simulink model "simulation17PDfract"  (R2025b)
settings: Solver=ode45  StartTime=0.0  StopTime=0.5  FixedStep=h  RelTol=1e-9
values from neighbouring files (symbols this model uses):
  h = 0.001    [run_3d_simbody_suite.m]    (also in run_all_simulations.m)
  kd = 1.0245    [run_3d_simbody_suite.m]
  kp = 16    [run_3d_simbody_suite.m]
  mu = 0.5308    [run_3d_simbody_suite.m]
  n = double(ceil(tf/h))    [run_3d_simbody_suite.m]    (also in run_all_simulations.m)
undefined symbols (not defined in the file or in its folder): X, Y, Z
libraries: sm_lib x327, nesl_utility x14, simulink x7, fod x3, checkpacklib x1
(part 8 of 8)

== system simulation17PDfract/RD_SM2/BrasParalelle1/BarreParalleles_2_RIGID/Pice4_Extremetees_1_RIGID ==
  ReferenceFrame : sm_lib/Frames and Transforms/Reference Frame
  Solid : sm_lib/Body Elements/File Solid  ExtGeomFileName=Pièce4_Extremetees_Défaut_sldprt.STL  UnitType=Custom  ExtGeomFileUnits=mm  StepReaderType=HEX  ExportConvexHullGeometry=off  InertiaType=Custom  Mass=0.0043409919402835973  MassUnits=kg  CenterOfMass=[-6.6394731011390018e-06 -1.3723999560385911 4.9969803448403587]  CenterOfMassUnits=mm  MomentsOfInertia=[0.22208105944838133 0.24049053699814107 0.066049415613599144]  MomentsOfInertiaUnits=kg*mm^2  ProductsOfInertia=[-0.022728057317176146 1.1398156711642886e-07 7.9844492116922665e-07]  ProductsOfInertiaUnits=kg*mm^2  BasedOnType=Density  Density=1000  DensityUnits=kg/(m^3)  DoExposeReferenceFrame=on  SerializedFrames=<Frames/>  GraphicType=FromGeometry  MarkerShape=Sphere  MarkerSize=10  MarkerSizeUnits=m  GraphicVisPropType=SimpleVisualProperties  GraphicDiffuseColor=[0.59999999999999998 0.59999999999999998 0.59999999999999998]  GraphicSpecularColor=[0.5 0.5 0.5 1.0]  GraphicAmbientColor=[0.15 0.15 0.15 1.0]  GraphicEmissiveColor=[0.0 0.0 0.0 1.0]  GraphicShininess=75  GraphicOpacity=1
  F : PMIOPort  Side=Left
  connections:
  Solid/RConn1 -- ReferenceFrame/RConn1 -- F/RConn1

== system simulation17PDfract/RD_SM2/BrasParalelle1/BarreParalleles_2_RIGID/Pice4_Extremetees_2_RIGID ==
  ReferenceFrame : sm_lib/Frames and Transforms/Reference Frame
  Solid : sm_lib/Body Elements/File Solid  ExtGeomFileName=Pièce4_Extremetees_Défaut_sldprt.STL  UnitType=Custom  ExtGeomFileUnits=mm  StepReaderType=HEX  ExportConvexHullGeometry=off  InertiaType=Custom  Mass=0.0043409919402835973  MassUnits=kg  CenterOfMass=[-6.6394731011390018e-06 -1.3723999560385911 4.9969803448403587]  CenterOfMassUnits=mm  MomentsOfInertia=[0.22208105944838133 0.24049053699814107 0.066049415613599144]  MomentsOfInertiaUnits=kg*mm^2  ProductsOfInertia=[-0.022728057317176146 1.1398156711642886e-07 7.9844492116922665e-07]  ProductsOfInertiaUnits=kg*mm^2  BasedOnType=Density  Density=1000  DensityUnits=kg/(m^3)  DoExposeReferenceFrame=on  SerializedFrames=<Frames/>  GraphicType=FromGeometry  MarkerShape=Sphere  MarkerSize=10  MarkerSizeUnits=m  GraphicVisPropType=SimpleVisualProperties  GraphicDiffuseColor=[0.59999999999999998 0.59999999999999998 0.59999999999999998]  GraphicSpecularColor=[0.5 0.5 0.5 1.0]  GraphicAmbientColor=[0.15 0.15 0.15 1.0]  GraphicEmissiveColor=[0.0 0.0 0.0 1.0]  GraphicShininess=75  GraphicOpacity=1
  F : PMIOPort  Side=Left
  connections:
  Solid/RConn1 -- ReferenceFrame/RConn1 -- F/RConn1

== system simulation17PDfract/RD_SM2/BrasParalelle1/BarreParalleles_2_RIGID/Pice4_Tube_1_RIGID ==
  ReferenceFrame : sm_lib/Frames and Transforms/Reference Frame
  Solid : sm_lib/Body Elements/File Solid  ExtGeomFileName=Pièce4_Tube_Défaut_sldprt.STL  UnitType=Custom  ExtGeomFileUnits=mm  StepReaderType=HEX  ExportConvexHullGeometry=off  InertiaType=Custom  Mass=0.0056953775725032503  MassUnits=kg  CenterOfMass=[-4.1460122344799134e-11 2.6332345173922464e-08 157.00037492761294]  CenterOfMassUnits=mm  MomentsOfInertia=[46.656669534748204 46.656784060773653 0.060513437161415502]  MomentsOfInertiaUnits=kg*mm^2  ProductsOfInertia=[4.4271388779002391e-06 -1.0344554341986986e-06 -6.5578304138838094e-07]  ProductsOfInertiaUnits=kg*mm^2  BasedOnType=Density  Density=1000  DensityUnits=kg/(m^3)  DoExposeReferenceFrame=on  SerializedFrames=<Frames/>  GraphicType=FromGeometry  MarkerShape=Sphere  MarkerSize=10  MarkerSizeUnits=m  GraphicVisPropType=SimpleVisualProperties  GraphicDiffuseColor=[1 1 1]  GraphicSpecularColor=[0.5 0.5 0.5 1.0]  GraphicAmbientColor=[0.15 0.15 0.15 1.0]  GraphicEmissiveColor=[0.0 0.0 0.0 1.0]  GraphicShininess=75  GraphicOpacity=1
  F : PMIOPort  Side=Left
  connections:
  Solid/RConn1 -- ReferenceFrame/RConn1 -- F/RConn1

== system simulation17PDfract/RD_SM2/BrasParalelle2/BarreParalleles_1_RIGID/Pice4_Extremetees_1_RIGID ==
  ReferenceFrame : sm_lib/Frames and Transforms/Reference Frame
  Solid : sm_lib/Body Elements/File Solid  ExtGeomFileName=Pièce4_Extremetees_Défaut_sldprt.STL  UnitType=Custom  ExtGeomFileUnits=mm  StepReaderType=HEX  ExportConvexHullGeometry=off  InertiaType=Custom  Mass=0.0043409919402835973  MassUnits=kg  CenterOfMass=[-6.6394731011390018e-06 -1.3723999560385911 4.9969803448403587]  CenterOfMassUnits=mm  MomentsOfInertia=[0.22208105944838133 0.24049053699814107 0.066049415613599144]  MomentsOfInertiaUnits=kg*mm^2  ProductsOfInertia=[-0.022728057317176146 1.1398156711642886e-07 7.9844492116922665e-07]  ProductsOfInertiaUnits=kg*mm^2  BasedOnType=Density  Density=1000  DensityUnits=kg/(m^3)  DoExposeReferenceFrame=on  SerializedFrames=<Frames/>  GraphicType=FromGeometry  MarkerShape=Sphere  MarkerSize=10  MarkerSizeUnits=m  GraphicVisPropType=SimpleVisualProperties  GraphicDiffuseColor=[0.59999999999999998 0.59999999999999998 0.59999999999999998]  GraphicSpecularColor=[0.5 0.5 0.5 1.0]  GraphicAmbientColor=[0.15 0.15 0.15 1.0]  GraphicEmissiveColor=[0.0 0.0 0.0 1.0]  GraphicShininess=75  GraphicOpacity=1
  F : PMIOPort  Side=Left
  connections:
  F/RConn1 -- ReferenceFrame/RConn1 -- Solid/RConn1

== system simulation17PDfract/RD_SM2/BrasParalelle2/BarreParalleles_1_RIGID/Pice4_Extremetees_2_RIGID ==
  ReferenceFrame : sm_lib/Frames and Transforms/Reference Frame
  Solid : sm_lib/Body Elements/File Solid  ExtGeomFileName=Pièce4_Extremetees_Défaut_sldprt.STL  UnitType=Custom  ExtGeomFileUnits=mm  StepReaderType=HEX  ExportConvexHullGeometry=off  InertiaType=Custom  Mass=0.0043409919402835973  MassUnits=kg  CenterOfMass=[-6.6394731011390018e-06 -1.3723999560385911 4.9969803448403587]  CenterOfMassUnits=mm  MomentsOfInertia=[0.22208105944838133 0.24049053699814107 0.066049415613599144]  MomentsOfInertiaUnits=kg*mm^2  ProductsOfInertia=[-0.022728057317176146 1.1398156711642886e-07 7.9844492116922665e-07]  ProductsOfInertiaUnits=kg*mm^2  BasedOnType=Density  Density=1000  DensityUnits=kg/(m^3)  DoExposeReferenceFrame=on  SerializedFrames=<Frames/>  GraphicType=FromGeometry  MarkerShape=Sphere  MarkerSize=10  MarkerSizeUnits=m  GraphicVisPropType=SimpleVisualProperties  GraphicDiffuseColor=[0.59999999999999998 0.59999999999999998 0.59999999999999998]  GraphicSpecularColor=[0.5 0.5 0.5 1.0]  GraphicAmbientColor=[0.15 0.15 0.15 1.0]  GraphicEmissiveColor=[0.0 0.0 0.0 1.0]  GraphicShininess=75  GraphicOpacity=1
  F : PMIOPort  Side=Left
  connections:
  F/RConn1 -- ReferenceFrame/RConn1 -- Solid/RConn1

== system simulation17PDfract/RD_SM2/BrasParalelle2/BarreParalleles_1_RIGID/Pice4_Tube_1_RIGID ==
  ReferenceFrame : sm_lib/Frames and Transforms/Reference Frame
  Solid : sm_lib/Body Elements/File Solid  ExtGeomFileName=Pièce4_Tube_Défaut_sldprt.STL  UnitType=Custom  ExtGeomFileUnits=mm  StepReaderType=HEX  ExportConvexHullGeometry=off  InertiaType=Custom  Mass=0.0056953775725032503  MassUnits=kg  CenterOfMass=[-4.1460122344799134e-11 2.6332345173922464e-08 157.00037492761294]  CenterOfMassUnits=mm  MomentsOfInertia=[46.656669534748204 46.656784060773653 0.060513437161415502]  MomentsOfInertiaUnits=kg*mm^2  ProductsOfInertia=[4.4271388779002391e-06 -1.0344554341986986e-06 -6.5578304138838094e-07]  ProductsOfInertiaUnits=kg*mm^2  BasedOnType=Density  Density=1000  DensityUnits=kg/(m^3)  DoExposeReferenceFrame=on  SerializedFrames=<Frames/>  GraphicType=FromGeometry  MarkerShape=Sphere  MarkerSize=10  MarkerSizeUnits=m  GraphicVisPropType=SimpleVisualProperties  GraphicDiffuseColor=[1 1 1]  GraphicSpecularColor=[0.5 0.5 0.5 1.0]  GraphicAmbientColor=[0.15 0.15 0.15 1.0]  GraphicEmissiveColor=[0.0 0.0 0.0 1.0]  GraphicShininess=75  GraphicOpacity=1
  F : PMIOPort  Side=Left
  connections:
  F/RConn1 -- ReferenceFrame/RConn1 -- Solid/RConn1

== system simulation17PDfract/RD_SM2/BrasParalelle2/BarreParalleles_2_RIGID/Pice4_Extremetees_1_RIGID ==
  ReferenceFrame : sm_lib/Frames and Transforms/Reference Frame
  Solid : sm_lib/Body Elements/File Solid  ExtGeomFileName=Pièce4_Extremetees_Défaut_sldprt.STL  UnitType=Custom  ExtGeomFileUnits=mm  StepReaderType=HEX  ExportConvexHullGeometry=off  InertiaType=Custom  Mass=0.0043409919402835973  MassUnits=kg  CenterOfMass=[-6.6394731011390018e-06 -1.3723999560385911 4.9969803448403587]  CenterOfMassUnits=mm  MomentsOfInertia=[0.22208105944838133 0.24049053699814107 0.066049415613599144]  MomentsOfInertiaUnits=kg*mm^2  ProductsOfInertia=[-0.022728057317176146 1.1398156711642886e-07 7.9844492116922665e-07]  ProductsOfInertiaUnits=kg*mm^2  BasedOnType=Density  Density=1000  DensityUnits=kg/(m^3)  DoExposeReferenceFrame=on  SerializedFrames=<Frames/>  GraphicType=FromGeometry  MarkerShape=Sphere  MarkerSize=10  MarkerSizeUnits=m  GraphicVisPropType=SimpleVisualProperties  GraphicDiffuseColor=[0.59999999999999998 0.59999999999999998 0.59999999999999998]  GraphicSpecularColor=[0.5 0.5 0.5 1.0]  GraphicAmbientColor=[0.15 0.15 0.15 1.0]  GraphicEmissiveColor=[0.0 0.0 0.0 1.0]  GraphicShininess=75  GraphicOpacity=1
  F : PMIOPort  Side=Left
  connections:
  F/RConn1 -- ReferenceFrame/RConn1 -- Solid/RConn1

== system simulation17PDfract/RD_SM2/BrasParalelle2/BarreParalleles_2_RIGID/Pice4_Extremetees_2_RIGID ==
  ReferenceFrame : sm_lib/Frames and Transforms/Reference Frame
  Solid : sm_lib/Body Elements/File Solid  ExtGeomFileName=Pièce4_Extremetees_Défaut_sldprt.STL  UnitType=Custom  ExtGeomFileUnits=mm  StepReaderType=HEX  ExportConvexHullGeometry=off  InertiaType=Custom  Mass=0.0043409919402835973  MassUnits=kg  CenterOfMass=[-6.6394731011390018e-06 -1.3723999560385911 4.9969803448403587]  CenterOfMassUnits=mm  MomentsOfInertia=[0.22208105944838133 0.24049053699814107 0.066049415613599144]  MomentsOfInertiaUnits=kg*mm^2  ProductsOfInertia=[-0.022728057317176146 1.1398156711642886e-07 7.9844492116922665e-07]  ProductsOfInertiaUnits=kg*mm^2  BasedOnType=Density  Density=1000  DensityUnits=kg/(m^3)  DoExposeReferenceFrame=on  SerializedFrames=<Frames/>  GraphicType=FromGeometry  MarkerShape=Sphere  MarkerSize=10  MarkerSizeUnits=m  GraphicVisPropType=SimpleVisualProperties  GraphicDiffuseColor=[0.59999999999999998 0.59999999999999998 0.59999999999999998]  GraphicSpecularColor=[0.5 0.5 0.5 1.0]  GraphicAmbientColor=[0.15 0.15 0.15 1.0]  GraphicEmissiveColor=[0.0 0.0 0.0 1.0]  GraphicShininess=75  GraphicOpacity=1
  F : PMIOPort  Side=Left
  connections:
  F/RConn1 -- ReferenceFrame/RConn1 -- Solid/RConn1

== system simulation17PDfract/RD_SM2/BrasParalelle2/BarreParalleles_2_RIGID/Pice4_Tube_1_RIGID ==
  ReferenceFrame : sm_lib/Frames and Transforms/Reference Frame
  Solid : sm_lib/Body Elements/File Solid  ExtGeomFileName=Pièce4_Tube_Défaut_sldprt.STL  UnitType=Custom  ExtGeomFileUnits=mm  StepReaderType=HEX  ExportConvexHullGeometry=off  InertiaType=Custom  Mass=0.0056953775725032503  MassUnits=kg  CenterOfMass=[-4.1460122344799134e-11 2.6332345173922464e-08 157.00037492761294]  CenterOfMassUnits=mm  MomentsOfInertia=[46.656669534748204 46.656784060773653 0.060513437161415502]  MomentsOfInertiaUnits=kg*mm^2  ProductsOfInertia=[4.4271388779002391e-06 -1.0344554341986986e-06 -6.5578304138838094e-07]  ProductsOfInertiaUnits=kg*mm^2  BasedOnType=Density  Density=1000  DensityUnits=kg/(m^3)  DoExposeReferenceFrame=on  SerializedFrames=<Frames/>  GraphicType=FromGeometry  MarkerShape=Sphere  MarkerSize=10  MarkerSizeUnits=m  GraphicVisPropType=SimpleVisualProperties  GraphicDiffuseColor=[1 1 1]  GraphicSpecularColor=[0.5 0.5 0.5 1.0]  GraphicAmbientColor=[0.15 0.15 0.15 1.0]  GraphicEmissiveColor=[0.0 0.0 0.0 1.0]  GraphicShininess=75  GraphicOpacity=1
  F : PMIOPort  Side=Left
  connections:
  F/RConn1 -- ReferenceFrame/RConn1 -- Solid/RConn1

== system simulation17PDfract/RD_SM2/BrasParalelle3/BarreParalleles_1_RIGID/Pice4_Extremetees_1_RIGID ==
  ReferenceFrame : sm_lib/Frames and Transforms/Reference Frame
  Solid : sm_lib/Body Elements/File Solid  ExtGeomFileName=Pièce4_Extremetees_Défaut_sldprt.STL  UnitType=Custom  ExtGeomFileUnits=mm  StepReaderType=HEX  ExportConvexHullGeometry=off  InertiaType=Custom  Mass=0.0043409919402835973  MassUnits=kg  CenterOfMass=[-6.6394731011390018e-06 -1.3723999560385911 4.9969803448403587]  CenterOfMassUnits=mm  MomentsOfInertia=[0.22208105944838133 0.24049053699814107 0.066049415613599144]  MomentsOfInertiaUnits=kg*mm^2  ProductsOfInertia=[-0.022728057317176146 1.1398156711642886e-07 7.9844492116922665e-07]  ProductsOfInertiaUnits=kg*mm^2  BasedOnType=Density  Density=1000  DensityUnits=kg/(m^3)  DoExposeReferenceFrame=on  SerializedFrames=<Frames/>  GraphicType=FromGeometry  MarkerShape=Sphere  MarkerSize=10  MarkerSizeUnits=m  GraphicVisPropType=SimpleVisualProperties  GraphicDiffuseColor=[0.59999999999999998 0.59999999999999998 0.59999999999999998]  GraphicSpecularColor=[0.5 0.5 0.5 1.0]  GraphicAmbientColor=[0.15 0.15 0.15 1.0]  GraphicEmissiveColor=[0.0 0.0 0.0 1.0]  GraphicShininess=75  GraphicOpacity=1
  F : PMIOPort  Side=Left
  connections:
  Solid/RConn1 -- ReferenceFrame/RConn1 -- F/RConn1

== system simulation17PDfract/RD_SM2/BrasParalelle3/BarreParalleles_1_RIGID/Pice4_Extremetees_2_RIGID ==
  ReferenceFrame : sm_lib/Frames and Transforms/Reference Frame
  Solid : sm_lib/Body Elements/File Solid  ExtGeomFileName=Pièce4_Extremetees_Défaut_sldprt.STL  UnitType=Custom  ExtGeomFileUnits=mm  StepReaderType=HEX  ExportConvexHullGeometry=off  InertiaType=Custom  Mass=0.0043409919402835973  MassUnits=kg  CenterOfMass=[-6.6394731011390018e-06 -1.3723999560385911 4.9969803448403587]  CenterOfMassUnits=mm  MomentsOfInertia=[0.22208105944838133 0.24049053699814107 0.066049415613599144]  MomentsOfInertiaUnits=kg*mm^2  ProductsOfInertia=[-0.022728057317176146 1.1398156711642886e-07 7.9844492116922665e-07]  ProductsOfInertiaUnits=kg*mm^2  BasedOnType=Density  Density=1000  DensityUnits=kg/(m^3)  DoExposeReferenceFrame=on  SerializedFrames=<Frames/>  GraphicType=FromGeometry  MarkerShape=Sphere  MarkerSize=10  MarkerSizeUnits=m  GraphicVisPropType=SimpleVisualProperties  GraphicDiffuseColor=[0.59999999999999998 0.59999999999999998 0.59999999999999998]  GraphicSpecularColor=[0.5 0.5 0.5 1.0]  GraphicAmbientColor=[0.15 0.15 0.15 1.0]  GraphicEmissiveColor=[0.0 0.0 0.0 1.0]  GraphicShininess=75  GraphicOpacity=1
  F : PMIOPort  Side=Left
  connections:
  Solid/RConn1 -- ReferenceFrame/RConn1 -- F/RConn1

== system simulation17PDfract/RD_SM2/BrasParalelle3/BarreParalleles_1_RIGID/Pice4_Tube_1_RIGID ==
  ReferenceFrame : sm_lib/Frames and Transforms/Reference Frame
  Solid : sm_lib/Body Elements/File Solid  ExtGeomFileName=Pièce4_Tube_Défaut_sldprt.STL  UnitType=Custom  ExtGeomFileUnits=mm  StepReaderType=HEX  ExportConvexHullGeometry=off  InertiaType=Custom  Mass=0.0056953775725032503  MassUnits=kg  CenterOfMass=[-4.1460122344799134e-11 2.6332345173922464e-08 157.00037492761294]  CenterOfMassUnits=mm  MomentsOfInertia=[46.656669534748204 46.656784060773653 0.060513437161415502]  MomentsOfInertiaUnits=kg*mm^2  ProductsOfInertia=[4.4271388779002391e-06 -1.0344554341986986e-06 -6.5578304138838094e-07]  ProductsOfInertiaUnits=kg*mm^2  BasedOnType=Density  Density=1000  DensityUnits=kg/(m^3)  DoExposeReferenceFrame=on  SerializedFrames=<Frames/>  GraphicType=FromGeometry  MarkerShape=Sphere  MarkerSize=10  MarkerSizeUnits=m  GraphicVisPropType=SimpleVisualProperties  GraphicDiffuseColor=[1 1 1]  GraphicSpecularColor=[0.5 0.5 0.5 1.0]  GraphicAmbientColor=[0.15 0.15 0.15 1.0]  GraphicEmissiveColor=[0.0 0.0 0.0 1.0]  GraphicShininess=75  GraphicOpacity=1
  F : PMIOPort  Side=Left
  connections:
  Solid/RConn1 -- ReferenceFrame/RConn1 -- F/RConn1

== system simulation17PDfract/RD_SM2/BrasParalelle3/BarreParalleles_2_RIGID/Pice4_Extremetees_1_RIGID ==
  ReferenceFrame : sm_lib/Frames and Transforms/Reference Frame
  Solid : sm_lib/Body Elements/File Solid  ExtGeomFileName=Pièce4_Extremetees_Défaut_sldprt.STL  UnitType=Custom  ExtGeomFileUnits=mm  StepReaderType=HEX  ExportConvexHullGeometry=off  InertiaType=Custom  Mass=0.0043409919402835973  MassUnits=kg  CenterOfMass=[-6.6394731011390018e-06 -1.3723999560385911 4.9969803448403587]  CenterOfMassUnits=mm  MomentsOfInertia=[0.22208105944838133 0.24049053699814107 0.066049415613599144]  MomentsOfInertiaUnits=kg*mm^2  ProductsOfInertia=[-0.022728057317176146 1.1398156711642886e-07 7.9844492116922665e-07]  ProductsOfInertiaUnits=kg*mm^2  BasedOnType=Density  Density=1000  DensityUnits=kg/(m^3)  DoExposeReferenceFrame=on  SerializedFrames=<Frames/>  GraphicType=FromGeometry  MarkerShape=Sphere  MarkerSize=10  MarkerSizeUnits=m  GraphicVisPropType=SimpleVisualProperties  GraphicDiffuseColor=[0.59999999999999998 0.59999999999999998 0.59999999999999998]  GraphicSpecularColor=[0.5 0.5 0.5 1.0]  GraphicAmbientColor=[0.15 0.15 0.15 1.0]  GraphicEmissiveColor=[0.0 0.0 0.0 1.0]  GraphicShininess=75  GraphicOpacity=1
  F : PMIOPort  Side=Left
  connections:
  Solid/RConn1 -- ReferenceFrame/RConn1 -- F/RConn1

== system simulation17PDfract/RD_SM2/BrasParalelle3/BarreParalleles_2_RIGID/Pice4_Extremetees_2_RIGID ==
  ReferenceFrame : sm_lib/Frames and Transforms/Reference Frame
  Solid : sm_lib/Body Elements/File Solid  ExtGeomFileName=Pièce4_Extremetees_Défaut_sldprt.STL  UnitType=Custom  ExtGeomFileUnits=mm  StepReaderType=HEX  ExportConvexHullGeometry=off  InertiaType=Custom  Mass=0.0043409919402835973  MassUnits=kg  CenterOfMass=[-6.6394731011390018e-06 -1.3723999560385911 4.9969803448403587]  CenterOfMassUnits=mm  MomentsOfInertia=[0.22208105944838133 0.24049053699814107 0.066049415613599144]  MomentsOfInertiaUnits=kg*mm^2  ProductsOfInertia=[-0.022728057317176146 1.1398156711642886e-07 7.9844492116922665e-07]  ProductsOfInertiaUnits=kg*mm^2  BasedOnType=Density  Density=1000  DensityUnits=kg/(m^3)  DoExposeReferenceFrame=on  SerializedFrames=<Frames/>  GraphicType=FromGeometry  MarkerShape=Sphere  MarkerSize=10  MarkerSizeUnits=m  GraphicVisPropType=SimpleVisualProperties  GraphicDiffuseColor=[0.59999999999999998 0.59999999999999998 0.59999999999999998]  GraphicSpecularColor=[0.5 0.5 0.5 1.0]  GraphicAmbientColor=[0.15 0.15 0.15 1.0]  GraphicEmissiveColor=[0.0 0.0 0.0 1.0]  GraphicShininess=75  GraphicOpacity=1
  F : PMIOPort  Side=Left
  connections:
  Solid/RConn1 -- ReferenceFrame/RConn1 -- F/RConn1

== system simulation17PDfract/RD_SM2/BrasParalelle3/BarreParalleles_2_RIGID/Pice4_Tube_1_RIGID ==
  ReferenceFrame : sm_lib/Frames and Transforms/Reference Frame
  Solid : sm_lib/Body Elements/File Solid  ExtGeomFileName=Pièce4_Tube_Défaut_sldprt.STL  UnitType=Custom  ExtGeomFileUnits=mm  StepReaderType=HEX  ExportConvexHullGeometry=off  InertiaType=Custom  Mass=0.0056953775725032503  MassUnits=kg  CenterOfMass=[-4.1460122344799134e-11 2.6332345173922464e-08 157.00037492761294]  CenterOfMassUnits=mm  MomentsOfInertia=[46.656669534748204 46.656784060773653 0.060513437161415502]  MomentsOfInertiaUnits=kg*mm^2  ProductsOfInertia=[4.4271388779002391e-06 -1.0344554341986986e-06 -6.5578304138838094e-07]  ProductsOfInertiaUnits=kg*mm^2  BasedOnType=Density  Density=1000  DensityUnits=kg/(m^3)  DoExposeReferenceFrame=on  SerializedFrames=<Frames/>  GraphicType=FromGeometry  MarkerShape=Sphere  MarkerSize=10  MarkerSizeUnits=m  GraphicVisPropType=SimpleVisualProperties  GraphicDiffuseColor=[1 1 1]  GraphicSpecularColor=[0.5 0.5 0.5 1.0]  GraphicAmbientColor=[0.15 0.15 0.15 1.0]  GraphicEmissiveColor=[0.0 0.0 0.0 1.0]  GraphicShininess=75  GraphicOpacity=1
  F : PMIOPort  Side=Left
  connections:
  Solid/RConn1 -- ReferenceFrame/RConn1 -- F/RConn1

== matlab function simulation17PDfract/fract PID2/frac_deriv/MATLAB Function ==
  data: u1 input; u2 input; u3 input; df output; clock input; q input; h input; n input
function df  = fcn(u1,u2,u3,clock,q,h,n)

df1 = 0;
df2 = 0;
df3 = 0;


cqj = zeros(1,501);

j = ceil(clock/h);
cqj(1,1) = 1;

for i = 1:j
    
    if i~=1
        cqj(i) = cqj(i-1)*(1-(1+q)/(i-1));
    end

    df1 = df1+h^-q*cqj(i)*u1(i);
    df2 = df2+h^-q*cqj(i)*u2(i);
    df3 = df3+h^-q*cqj(i)*u3(i);
end

df = [df1 df2 df3];

== matlab function simulation17PDfract/MATLAB Function6 ==
  data: P input; x output; y output; z output
function [x,y,z] = demux(P)
x = P(1,1);
y = P(1,2);
z = P(1,3);

== matlab function simulation17PDfract/RD_SM2/adaptation ==
  data: alpha input; Theta output; dalpha input; dTheta output
function [Theta,dTheta]= fcn(alpha,dalpha)
%RQ : l'angle alpha est decalee de shift = -0.0651 red (problemme simmechanics)
Theta = -12*(alpha - 0.0651*[1;1;1]) ;
dTheta = -12*dalpha ;

== matlab function simulation17PDfract/trajectoire/MATLAB Function1 ==
  data: P output; p input; t input; dP output; ddP output
function [P,dP,ddP]  = trajectoire(p,t)


A=0.25;
B=0.06;
D=pi*sqrt((A^2+B^2)/2);



Xdes=0.25-A*(1-cos(pi*(t)/(p*D)));
Ydes=0*t;
Zdes=-0.43+B*sin(pi*(t)/(p*D));

dXdes=-A*pi/(p*D)*(sin(pi*(t)/(p*D)));
dYdes=0*t;
dZdes=B*pi/(p*D)*cos(pi*(t)/(p*D));

ddXdes=A*pi/(p*D)*pi/(p*D)*cos(pi*(t)/(p*D));
ddYdes=0*t;
ddZdes=-B*pi/(p*D)*pi/(p*D)*sin(pi*(t)/(p*D));

% Xdes=-0.25+A*(1-cos(pi*t/(p*D)));
% Ydes=0*t;
% Zdes=-0.43+B*sin(pi*t/(p*D));

P = [Xdes,Ydes,Zdes];
dP = [dXdes,dYdes,dZdes];
ddP = [ddXdes,ddYdes,ddZdes];

end

== matlab function simulation17PDfract/MATLAB Function ==
  data: alpha input; P output; data input
function P  = MGD(alpha, data)

phi = [0 2*pi/3 4*pi/3];
l1 = 0.205;
l2 = 0.380;
r = 0.15-0.024;

D = zeros(1,3);
E = zeros(1,3);
F = zeros(1,3);
G = zeros(1,3);

for i=1:3
   D(i)=-l2^2+l1^2+r^2+2*r*l1*cos(alpha(i));
   E(i)=2*(r+l1*cos(alpha(i)))*cos(phi(i));
   F(i)=2*(r+l1*cos(alpha(i)))*sin(phi(i));
   G(i)=-2*l1*sin(alpha(i))  ;
end
% H1 = -(E(3)-E(1))*(G(2)-G(1))+(G(3)-G(1))*(E(2)-E(1));
% H2 = -(F(3)-F(1))*(E(2)-E(1))+(E(3)-E(1))*(F(2)-F(1));
% H3 = -(D(3)-D(1))*(E(2)-E(1))+(E(3)-E(1))*(D(2)-D(1));
% H4 = (D(3)-D(1))*(F(2)-F(1))-(F(3)-F(1))*(D(1)-D(2));
% H5 = -(G(3)-G(1))*(F(2)-F(1))-(F(3)-F(1))*(G(1)-G(2));

H1 = E(1)*G(2)-E(1)*G(3)-E(2)*G(1)+E(2)*G(3)+E(3)*G(1)-E(3)*G(2);
H2 = E(1)*(-F(2)+F(3))+E(2)*(F(1)-F(3))+E(3)*(-F(1)+F(2));
H3 = E(1)*(-D(2)+D(3))+E(2)*(D(1)-D(3))+E(3)*(-D(1)+D(2));
H4 = F(1)*(D(2)-D(3))+F(2)*(-D(1)+D(3))+F(3)*(D(1)-D(2));
H5 = F(1)*(-G(2)+G(3))+F(2)*(G(1)-G(3))+F(3)*(-G(1)+G(2));

L = ((H5^2+H1^2)/(H2^2))+1;
M = 2*(H5*H4+H1*H3)/(H2^2)-(H5*E(1)+H1*F(1))/H2-G(1);
N = (H4^2+H3^2)/H2^2-(H4*E(1)+H3*F(1))/H2+D(1);
Z = min((-M+sqrt(abs(M^2-4*L*N)))/(2*L),(-M-sqrt(abs(M^2-4*L*N)))/(2*L));
X = Z*(H5/H2)+(H4/H2);
Y = Z*(H1/H2)+(H3/H2);

X = double(X);
Y = double(Y);
Z = double(Z);

P = [X,Y,Z];

== matlab function simulation17PDfract/model inverse/MATLAB Function4 ==
  data: alpha input; ddalpha output; dalpha input; P input; dP input; ddP input
function ddalpha = MAI(alpha,dalpha,P,dP,ddP)

phi = [0 2*pi/3 4*pi/3];
l1 = 0.205;
r = 0.15-0.024;

% documentation 0

% rotation matrix
R1 = [cos(phi(1)) -sin(phi(1)) 0;sin(phi(1)) cos(phi(1)) 0;0 0 1];
R2 = [cos(phi(2)) -sin(phi(2)) 0;sin(phi(2)) cos(phi(2)) 0;0 0 1]; 
R3 = [cos(phi(3)) -sin(phi(3)) 0;sin(phi(3)) cos(phi(3)) 0;0 0 1]; 

% eq 4.4
s1 = [P(1);P(2);P(3)]-R1*([r;0;0]+[l1*cos(alpha(1));0;l1*sin(alpha(1))]);    
s2 = [P(1);P(2);P(3)]-R2*([r;0;0]+[l1*cos(alpha(2));0;l1*sin(alpha(2))]); 
s3 = [P(1);P(2);P(3)]-R3*([r;0;0]+[l1*cos(alpha(3));0;l1*sin(alpha(3))]); 

% eq 4.9
b1 = R1*[-l1*sin(alpha(1));0;l1*cos(alpha(1))];
b2 = R2*[-l1*sin(alpha(2));0;l1*cos(alpha(2))];
b3 = R3*[-l1*sin(alpha(3));0;l1*cos(alpha(3))];

% eq 4.8
ds1 = [dP(1);dP(2);dP(3)]-R1*[-l1*sin(alpha(1));0;l1*cos(alpha(1))]*dalpha(1);
ds2 = [dP(1);dP(2);dP(3)]-R2*[-l1*sin(alpha(2));0;l1*cos(alpha(2))]*dalpha(2);
ds3 = [dP(1);dP(2);dP(3)]-R3*[-l1*sin(alpha(3));0;l1*cos(alpha(3))]*dalpha(3);

db1 = R1*[-l1*cos(alpha(1));0;-l1*sin(alpha(1))]*dalpha(1);
db2 = R2*[-l1*cos(alpha(2));0;-l1*sin(alpha(2))]*dalpha(2);
db3 = R3*[-l1*cos(alpha(3));0;-l1*sin(alpha(3))]*dalpha(3);


% eq 4.15
ddalpha = (inv([s1'*b1 0 0;0 s2'*b2 0;0 0 s3'*b3])*([s1';s2';s3']*ddP'+[ds1';ds2';ds3']*dP'-[ds1'*b1+s1'*db1 0 0;0 ds2'*b2+s2'*db2 0;0 0 ds3'*b3+s3'*db3]*dalpha'))';
if isnan(ddalpha)
    ddalpha = zeros(1,3);
end

== matlab function simulation17PDfract/MATLAB Function2 ==
  data: u1 input; alpha output; u2 input; u3 input
function alpha = mux(u1,u2,u3)

alpha = [u1 u2 u3];

== matlab function simulation17PDfract/fract PID1/frac_deriv/MATLAB Function ==
  data: u1 input; u2 input; u3 input; df output; clock input; q input; h input; n input
function df  = fcn(u1,u2,u3,clock,q,h,n)

df1 = 0;
df2 = 0;
df3 = 0;

f1 = zeros(1,50001);
f2 = zeros(1,50001);
f3 = zeros(1,50001);
cqj = zeros(1,50001);

j = ceil(clock/h);
cqj(1,1) = 1;

for i = 1:j
f1(i) = u1(j-i+1);
f2(i) = u2(j-i+1);
f3(i) = u3(j-i+1);
    if i~=1
        cqj(i) = cqj(i-1)*(1-(1+q)/(i-1));
    end
end

for i = 1:j
    df1 = df1+h^-q*cqj(i)*f1(j-i+1);
    df2 = df2+h^-q*cqj(i)*f2(j-i+1);
    df3 = df3+h^-q*cqj(i)*f3(j-i+1);
end

df = [df1 df2 df3];

== matlab function simulation17PDfract/MATLAB Function1 ==
  data: u1 input; alpha output; u2 input; u3 input
function alpha = mux(u1,u2,u3)

alpha = [u1 u2 u3];

== matlab function simulation17PDfract/MATLAB Function4 ==
  data: P input; x output; y output; z output
function [x,y,z] = demux(P)
x = P(1,1);
y = P(1,2);
z = P(1,3);

== matlab function simulation17PDfract/model inverse/MATLAB Function5 ==
  data: P input; dP input; dalpha output; stepTime input
function dalpha = MCI(P,dP,stepTime)

phi = [0 2*pi/3 4*pi/3];
l1 = 0.205;
l2 = 0.380;
r = 0.15-0.024;

X = P(1);
Y = P(2);
Z = P(3);

dX = dP(1);
dY = dP(2);
dZ = dP(3);

A = zeros(1,3);
B = 2*(Z+dZ*stepTime)*l1;
C = zeros(1,3);

for i=1:3
A(i) = 2*r*l1-2*(X+dX*stepTime)*l1*cos(phi(i))-2*(Y+dY*stepTime)*l1*sin(phi(i));
C(i) = l2^2-l1^2-r^2-(X+dX*stepTime)^2-(Y+dY*stepTime)^2-(Z+dZ*stepTime)^2+2*(X+dX*stepTime)*r*cos(phi(i))+2*(Y+dY*stepTime)*r*sin(phi(i));    
end

alpha1 = zeros(1,3);
for i=1:3
    alpha1(i) =  2*atan( (2*B+sqrt(abs(4*B^2+4*(A(i)+C(i))*(A(i)-C(i)))))/(2*(A(i)+C(i))));
    alpha1(i) = double(alpha1(i));
end

A = zeros(1,3);
B = 2*Z*l1;
C = zeros(1,3);

for i=1:3
A(i) = 2*r*l1-2*X*l1*cos(phi(i))-2*Y*l1*sin(phi(i));
C(i) = l2^2-l1^2-r^2-X^2-Y^2-Z^2+2*X*r*cos(phi(i))+2*Y*r*sin(phi(i));    
end

alpha0 = zeros(1,3);
for i=1:3
    alpha0(i) =  2*atan( (2*B+sqrt(abs(4*B^2+4*(A(i)+C(i))*(A(i)-C(i)))))/(2*(A(i)+C(i))));
    alpha0(i) = double(alpha0(i));
end

dalpha = zeros(1,3);
for i=1:3
    dalpha(i) = double((alpha1(i)-alpha0(i))/stepTime);
end
if isnan(dalpha)
    dalpha = zeros(1,3);
end

== matlab function simulation17PDfract/model inverse/MATLAB Function6 ==
  data: P input; alpha output
function alpha = MGI(P)
phi = [0 2*pi/3 4*pi/3];
l1 = 0.205;
l2 = 0.380;
r = 0.15-0.024;
X = P(1,1);
Y = P(1,2);
Z = P(1,3);

A = zeros(1,3);
B = 2*Z*l1;
C = zeros(1,3);

for i=1:3
A(i) = 2*r*l1-2*X*l1*cos(phi(i))-2*Y*l1*sin(phi(i));
C(i) = l2^2-l1^2-r^2-X^2-Y^2-Z^2+2*X*r*cos(phi(i))+2*Y*r*sin(phi(i));    
end

alpha = zeros(1,3);
for i=1:3
    alpha(i) =  2*atan( (2*B+sqrt(abs(4*B^2+4*(A(i)+C(i))*(A(i)-C(i)))))/(2*(A(i)+C(i))));
    alpha(i) = double(alpha(i));
end
